simulink model "lab5_2b"  (R2019b)
settings: Solver=VariableStepAuto  StartTime=0.0  StopTime=10.0  RelTol=1e-3
settings Model: Creator=82354  LastModifiedBy=82354

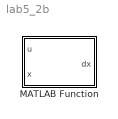
== system lab5_2b ==
  MATLAB Function : MATLAB Function  TreatAsAtomicUnit=on

== matlab function lab5_2b/MATLAB Function ==
  data: u input; dx output; x input
function dx = fcn(u,x)




dx = u+x;
